simulink model "mophongPID"  (Simulink 8.0)
settings: Solver=ode3  StartTime=0.0  StopTime=8  FixedStep=0.01  RelTol=1e-2
values from neighbouring files (symbols this model uses):
  g = 9.81    [PID_thayLuu.m]    (also in thongsohethong.m)
  K1 = Rm*Jm*L/Km/Kg/d+J1    (= 0.103280702164)    [PID_thayLuu.m]    (also in thongsohethong.m)
  K2 = L/d*(Km*Kb/Rm+Kb+Rm*Bm/Km/Kg)    (= 0.430559496256)    [PID_thayLuu.m]    (also in thongsohethong.m)
  K3 = 1+Km/Rm    (= 1.01514285714)    [PID_thayLuu.m]    (also in thongsohethong.m)
  K4 = 7/5    (= 1.4)    [PID_thayLuu.m]    (also in thongsohethong.m)
  Kd1 = par(bestchrom,3)-1000    [pidGA.m]
  Kd2 = par(bestchrom,6)-1000    [pidGA.m]
  Ki1 = par(bestchrom,2)-1000    [pidGA.m]
  Ki2 = par(bestchrom,5)-1000    [pidGA.m]
  Kp1 = par(bestchrom,1)-1000    [pidGA.m]
  Kp2 = par(bestchrom,4)-1000    [pidGA.m]
  L = 0.55    [PID_thayLuu.m]    (also in thongsohethong.m)
  m = 43.56*10^-3    (= 0.04356)    [PID_thayLuu.m]    (also in thongsohethong.m)
  M = 346.6*10^-3    (= 0.3466)    [PID_thayLuu.m]    (also in thongsohethong.m)
  x1_init = 0    [PID_thayLuu.m]    (also in thongsohethong.m = 0.02)
  x2_init = 0    [PID_thayLuu.m]    (also in thongsohethong.m)
  x3_init = 0    [PID_thayLuu.m]    (also in thongsohethong.m = 0.01)
  x4_init = 0    [PID_thayLuu.m]    (also in thongsohethong.m)
settings Model: Creator=KHACH  LastModifiedBy=Admin
settings SolverCC: ZeroCrossAlgorithm=Adaptive
settings DataIOCC: SignalLoggingSaveFormat=ModelDataLogs
settings DebuggingCC: FcnCallInpInsideContextMsg=UseLocalSettings  StrictBusMsg=Warning
settings GRTTargetCC: CombineOutputUpdateFcns=off  GRTInterface=on

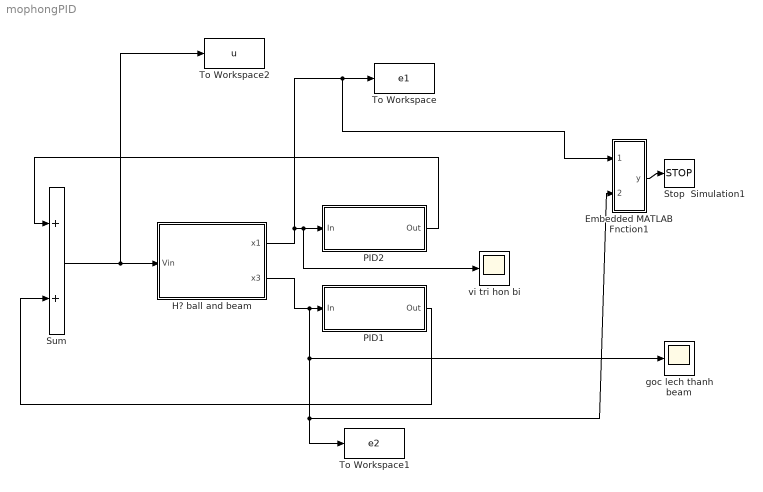
== system mophongPID ==
  Embedded MATLAB Fnction1 : MATLAB Function  TreatAsAtomicUnit=on
  H? ball and beam : Subsystem
  PID1 : Subsystem
  PID2 : Subsystem
  Stop  Simulation1 : Stop
  Sum : Sum
  To Workspace : ToWorkspace  VariableName=e1  SampleTime=-1
  To Workspace1 : ToWorkspace  VariableName=e2  SampleTime=-1
  To Workspace2 : ToWorkspace  VariableName=u  SampleTime=-1
  goc lech thanh beam : Scope
      settings: SaveName=ScopeData5
  vi tri hon bi : Scope
      settings: TimeRange=40  YMin=-0.1  YMax=0.225  SaveName=ScopeData4
  wires:
  Sum/1 -> To Workspace2/1, H? ball and beam/1(Vin)
  PID2/1(Out) -> Sum/1
  PID1/1(Out) -> Sum/2
  H? ball and beam/1(x1) -> Embedded MATLAB Fnction1/1(e1), To Workspace/1, vi tri hon bi/1, PID2/1(In)
  Embedded MATLAB Fnction1/1(y) -> Stop  Simulation1/1
  H? ball and beam/2(x3) -> Embedded MATLAB Fnction1/2(e2), To Workspace1/1, goc lech thanh beam/1, PID1/1(In)

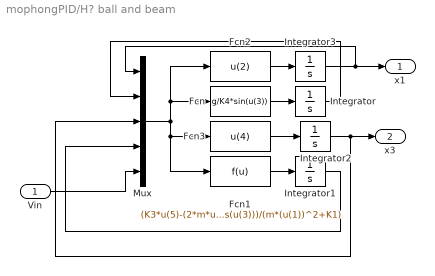
== system mophongPID/H? ball and beam ==
  Vin : Inport
  Fcn : Fcn  Expr=g/K4*sin(u(3))
  Fcn1 : Fcn  Expr=(K3*u(5)-(2*m*u(1)*u(2)+K2)*u(4)-(m*g*u(1)+L/2*M*g)*cos(u(3)))/(m*(u(1))^2+K1)
  Fcn2 : Fcn  Expr=u(2)
  Fcn3 : Fcn  Expr=u(4)
  Integrator : Integrator  InitialCondition=x2_init
  Integrator1 : Integrator  InitialCondition=x4_init
  Integrator2 : Integrator  InitialCondition=x3_init
  Integrator3 : Integrator  InitialCondition=x1_init
  Mux : Mux  Inputs=5
  x1 : Outport
  x3 : Outport  Port=2
  wires:
  Vin/1 -> Mux/5
  Mux/1 -> Fcn1/1, Fcn3/1, Fcn/1, Fcn2/1
  Fcn/1 -> Integrator/1
  Fcn1/1 -> Integrator1/1
  Fcn2/1 -> Integrator3/1
  Fcn3/1 -> Integrator2/1
  Integrator3/1 -> x1/1, Mux/1
  Integrator/1 -> Mux/2
  Integrator2/1 -> x3/1, Mux/3
  Integrator1/1 -> Mux/4

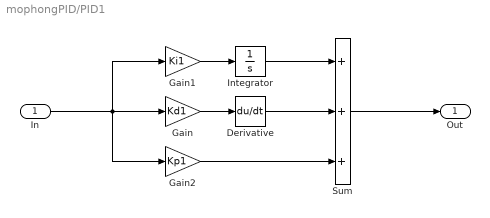
== system mophongPID/PID1 ==
  In : Inport
  Derivative : Derivative
  Gain : Gain  Gain=Kd1
  Gain1 : Gain  Gain=Ki1
  Gain2 : Gain  Gain=Kp1
  Integrator : Integrator
  Sum : Sum  Inputs=+++
  Out : Outport
  wires:
  Sum/1 -> Out/1
  Derivative/1 -> Sum/2
  Gain/1 -> Derivative/1
  Integrator/1 -> Sum/1
  Gain1/1 -> Integrator/1
  In/1 -> Gain2/1, Gain1/1, Gain/1
  Gain2/1 -> Sum/3

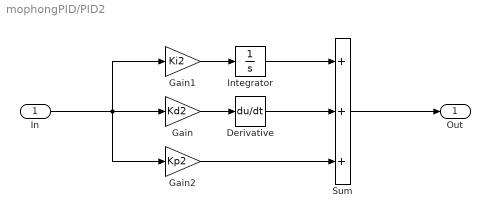
== system mophongPID/PID2 ==
  In : Inport
  Derivative : Derivative
  Gain : Gain  Gain=Kd2
  Gain1 : Gain  Gain=Ki2
  Gain2 : Gain  Gain=Kp2
  Integrator : Integrator
  Sum : Sum  Inputs=+++
  Out : Outport
  wires:
  Sum/1 -> Out/1
  Derivative/1 -> Sum/2
  Gain/1 -> Derivative/1
  Integrator/1 -> Sum/1
  Gain1/1 -> Integrator/1
  In/1 -> Gain2/1, Gain1/1, Gain/1
  Gain2/1 -> Sum/3

== matlab function Embedded MATLAB Fnction1 ==
  data: e1 input double; y output double; e2 input double
function y = fcn(e1,e2)
if (abs(e1)>(3))||(abs(e2)>(3))
    y=1;
else
    y=0;
end
